simulink model "teach_from_joints"  (R2021a)
settings: Solver=FixedStepAuto  StartTime=0.0  StopTime=1000  FixedStep=SAMPLE_TIME  RelTol=1e-3
values from neighbouring files (symbols this model uses):
  dh_a = dh_list(:,3)    [move_joints_setup.m]
  dh_alpha = dh_list(:,4)    [move_joints_setup.m]
  dh_d = dh_list(:,2)+[0 0 0 0 0 length_f2t]'    [move_joints_setup.m]
  dh_theta_offset = dh_list(:,1)    [move_joints_setup.m]
  init_position = [274.5 0 543.1-138]    [move_joints_setup.m]
  initial_q = [0, 0, 0, 0, pi/2, 0]    [move_joints_setup.m]
  SAMPLE_TIME = 0.004    [move_joints_setup.m]
  theta_acc_max = theta_vel_max*2    [move_joints_setup.m]
  theta_max = [180,	80, 	70,     180,	110,	360]*pi/180    [move_joints_setup.m]
  theta_min = [-180,	-120,     -100,	-195,	-120,	-360]*pi/180    [move_joints_setup.m]
  theta_vel_max = [15, 10, 10, 40, 40, 40]*pi/180    [move_joints_setup.m]
undefined symbols (not defined in the file or in its folder): Px, Py, Pz, X, Y, Z
libraries: sm_lib x70, simulink x12, nesl_utility x11, dspswit3 x3, simulink_extras x2, sldrtlib x1, aerolibanimutils x1
(part 2 of 3)

== system teach_from_joints/Virtual_Robot_Subsystem/link_5 ==
  Inertia : sm_lib/Body Elements/Inertia  InertiaType=Custom  Mass=0.686166613628173  MassUnits=kg  CenterOfMass=[0, 0, 0]  CenterOfMassUnits=m  MomentsOfInertia=[0.00132263212499977, 0.000588220900408187, 0.00129230706392879]  MomentsOfInertiaUnits=kg*m^2  ProductsOfInertia=[9.33973775010868e-07, 6.88476103717453e-07, 5.90361537979662e-07]  ProductsOfInertiaUnits=kg*m^2  GraphicType=Marker  MarkerShape=Inertia  MarkerSize=20  GraphicVisPropType=SimpleVisualProperties  GraphicDiffuseColor=[0.5 0.5 0.5]  GraphicSpecularColor=[0.5 0.5 0.5 1.0]  GraphicAmbientColor=[0.15 0.15 0.15 1.0]  GraphicEmissiveColor=[0.0 0.0 0.0 1.0]  GraphicShininess=75  GraphicOpacity=1.0
  InertiaOriginTransform : sm_lib/Frames and Transforms/Rigid Transform  TranslationMethod=Cartesian  TranslationStandardOffset=0  TranslationLengthUnit=m  TranslationStandardAxis=+Z  TranslationCartesianOffset=[-0.0411790220693793, -0.0218038179681588, 5.10804574672119e-05]  TranslationROffset=0  TranslationROffsetUnits=m  TranslationZOffset=0  TranslationZOffsetUnits=m  TranslationThetaOffset=0  TranslationThetaOffsetUnits=deg  RotationMethod=RotationSequence  RotationAngleUnits=deg  RotationStandardAxis=+Z  RotationAngle=0.0  RotationArbitraryAxis=[0 0 1]  FollAlignAxisA=+X  BaseAlignAxisA=+Y  FollAlignAxisB=+Y  BaseAlignAxisB=+Z  RotationSequenceAxes=BaseAxes  RotationSequence=XYZ  RotationSequenceAngles=[0, 0, 0]  RotationSequenceAnglesUnits=rad  RotationMatrix=[1 0 0; 0 1 0; 0 0 1]
  ReferenceFrame : sm_lib/Frames and Transforms/Reference Frame
  Visual : sm_lib/Body Elements/File Solid  ExtGeomFileName=D:\matlab\tools\Mytool\Links-RT\MX\link_5.STL  UnitType=Custom  ExtGeomFileUnits=m  StepReaderType=HEX  ExportConvexHullGeometry=off  InertiaType=Custom  Mass=0  MassUnits=kg  CenterOfMass=[0, 0, 0]  CenterOfMassUnits=m  MomentsOfInertia=[0, 0, 0]  MomentsOfInertiaUnits=kg*m^2  ProductsOfInertia=[0, 0, 0]  ProductsOfInertiaUnits=kg*m^2  BasedOnType=Density  Density=1000  DensityUnits=kg/m^3  DoExposeReferenceFrame=on  SerializedFrames=<Frames/>  GraphicType=FromGeometry  MarkerShape=Sphere  MarkerSize=10  GraphicVisPropType=SimpleVisualProperties  GraphicDiffuseColor=[0.6 0.0 0.6]  GraphicSpecularColor=[0.5 0.5 0.5 1.0]  GraphicAmbientColor=[0.15 0.15 0.15 1.0]  GraphicEmissiveColor=[0.0 0.0 0.0 1.0]  GraphicShininess=75  GraphicOpacity=1
  VisualOriginTransform : sm_lib/Frames and Transforms/Rigid Transform  TranslationMethod=Cartesian  TranslationStandardOffset=0  TranslationLengthUnit=m  TranslationStandardAxis=+Z  TranslationCartesianOffset=[0, 0, 0]  TranslationROffset=0  TranslationROffsetUnits=m  TranslationZOffset=0  TranslationZOffsetUnits=m  TranslationThetaOffset=0  TranslationThetaOffsetUnits=deg  RotationMethod=RotationSequence  RotationAngleUnits=deg  RotationStandardAxis=+Z  RotationAngle=0.0  RotationArbitraryAxis=[0 0 1]  FollAlignAxisA=+X  BaseAlignAxisA=+Y  FollAlignAxisB=+Y  BaseAlignAxisB=+Z  RotationSequenceAxes=BaseAxes  RotationSequence=XYZ  RotationSequenceAngles=[0, 0, 0]  RotationSequenceAnglesUnits=rad  RotationMatrix=[1 0 0; 0 1 0; 0 0 1]
  joint_5_AxisInvTransform : sm_lib/Frames and Transforms/Rigid Transform  TranslationMethod=Cartesian  TranslationStandardOffset=0  TranslationLengthUnit=m  TranslationStandardAxis=+Z  TranslationCartesianOffset=[0, 0, 0]  TranslationROffset=0  TranslationROffsetUnits=m  TranslationZOffset=0  TranslationZOffsetUnits=m  TranslationThetaOffset=0  TranslationThetaOffsetUnits=deg  RotationMethod=ArbitraryAxis  RotationAngleUnits=rad  RotationStandardAxis=+Z  RotationAngle=1.571333286617217  RotationArbitraryAxis=[0.0006852597403183663, 0.9999996210465608, 0]  FollAlignAxisA=+X  BaseAlignAxisA=+Y  FollAlignAxisB=+Y  BaseAlignAxisB=+Z  RotationSequenceAxes=FollowerAxes  RotationSequence=XYX  RotationSequenceAngles=[0 0 0]  RotationSequenceAnglesUnits=deg  RotationMatrix=[1 0 0; 0 1 0; 0 0 1]
  joint_6_AxisTransform : sm_lib/Frames and Transforms/Rigid Transform  TranslationMethod=Cartesian  TranslationStandardOffset=0  TranslationLengthUnit=m  TranslationStandardAxis=+Z  TranslationCartesianOffset=[0, 0, 0]  TranslationROffset=0  TranslationROffsetUnits=m  TranslationZOffset=0  TranslationZOffsetUnits=m  TranslationThetaOffset=0  TranslationThetaOffsetUnits=deg  RotationMethod=ArbitraryAxis  RotationAngleUnits=rad  RotationStandardAxis=+Z  RotationAngle=1.569925857218851  RotationArbitraryAxis=[0.9999993866728818, -0.0006847895799997227, 0]  FollAlignAxisA=+X  BaseAlignAxisA=+Y  FollAlignAxisB=+Y  BaseAlignAxisB=+Z  RotationSequenceAxes=FollowerAxes  RotationSequence=XYX  RotationSequenceAngles=[0 0 0]  RotationSequenceAnglesUnits=deg  RotationMatrix=[1 0 0; 0 1 0; 0 0 1]
  joint_6_OriginTransform : sm_lib/Frames and Transforms/Rigid Transform  TranslationMethod=Cartesian  TranslationStandardOffset=0  TranslationLengthUnit=m  TranslationStandardAxis=+Z  TranslationCartesianOffset=[-0.041164, -0.10196, 6.9996e-05]  TranslationROffset=0  TranslationROffsetUnits=m  TranslationZOffset=0  TranslationZOffsetUnits=m  TranslationThetaOffset=0  TranslationThetaOffsetUnits=deg  RotationMethod=RotationSequence  RotationAngleUnits=deg  RotationStandardAxis=+Z  RotationAngle=0.0  RotationArbitraryAxis=[0 0 1]  FollAlignAxisA=+X  BaseAlignAxisA=+Y  FollAlignAxisB=+Y  BaseAlignAxisB=+Z  RotationSequenceAxes=BaseAxes  RotationSequence=XYZ  RotationSequenceAngles=[0, 0, 0]  RotationSequenceAnglesUnits=rad  RotationMatrix=[1 0 0; 0 1 0; 0 0 1]
  F : PMIOPort  Side=Left
  F1 : PMIOPort  Port=2  Side=Right
  connections:
  Inertia/RConn1 -- InertiaOriginTransform/RConn1
  ReferenceFrame/RConn1 -- InertiaOriginTransform/LConn1 -- joint_5_AxisInvTransform/LConn1 -- joint_6_OriginTransform/LConn1 -- VisualOriginTransform/LConn1
  Visual/RConn1 -- VisualOriginTransform/RConn1
  joint_5_AxisInvTransform/RConn1 -- F/RConn1
  joint_6_AxisTransform/RConn1 -- F1/RConn1
  joint_6_AxisTransform/LConn1 -- joint_6_OriginTransform/RConn1

== system teach_from_joints/Virtual_Robot_Subsystem/link_6 ==
  Inertia : sm_lib/Body Elements/Inertia  InertiaType=Custom  Mass=0.0837748471575824  MassUnits=kg  CenterOfMass=[0, 0, 0]  CenterOfMassUnits=m  MomentsOfInertia=[2.37096430738442e-05, 3.68399701824941e-05, 2.31857885737575e-05]  MomentsOfInertiaUnits=kg*m^2  ProductsOfInertia=[7.52372333523442e-08, 1.62958387540116e-10, 8.749655143078051e-09]  ProductsOfInertiaUnits=kg*m^2  GraphicType=Marker  MarkerShape=Inertia  MarkerSize=20  GraphicVisPropType=SimpleVisualProperties  GraphicDiffuseColor=[0.5 0.5 0.5]  GraphicSpecularColor=[0.5 0.5 0.5 1.0]  GraphicAmbientColor=[0.15 0.15 0.15 1.0]  GraphicEmissiveColor=[0.0 0.0 0.0 1.0]  GraphicShininess=75  GraphicOpacity=1.0
  InertiaOriginTransform : sm_lib/Frames and Transforms/Rigid Transform  TranslationMethod=Cartesian  TranslationStandardOffset=0  TranslationLengthUnit=m  TranslationStandardAxis=+Z  TranslationCartesianOffset=[-1.49769939650213e-05, -0.0138878614398256, -0.000131426803611889]  TranslationROffset=0  TranslationROffsetUnits=m  TranslationZOffset=0  TranslationZOffsetUnits=m  TranslationThetaOffset=0  TranslationThetaOffsetUnits=deg  RotationMethod=RotationSequence  RotationAngleUnits=deg  RotationStandardAxis=+Z  RotationAngle=0.0  RotationArbitraryAxis=[0 0 1]  FollAlignAxisA=+X  BaseAlignAxisA=+Y  FollAlignAxisB=+Y  BaseAlignAxisB=+Z  RotationSequenceAxes=BaseAxes  RotationSequence=XYZ  RotationSequenceAngles=[0, 0, 0]  RotationSequenceAnglesUnits=rad  RotationMatrix=[1 0 0; 0 1 0; 0 0 1]
  ReferenceFrame : sm_lib/Frames and Transforms/Reference Frame
  Visual : sm_lib/Body Elements/File Solid  ExtGeomFileName=D:\matlab\tools\Mytool\Links-RT\MX\link_6.STL  UnitType=Custom  ExtGeomFileUnits=m  StepReaderType=HEX  ExportConvexHullGeometry=off  InertiaType=Custom  Mass=0  MassUnits=kg  CenterOfMass=[0, 0, 0]  CenterOfMassUnits=m  MomentsOfInertia=[0, 0, 0]  MomentsOfInertiaUnits=kg*m^2  ProductsOfInertia=[0, 0, 0]  ProductsOfInertiaUnits=kg*m^2  BasedOnType=Density  Density=1000  DensityUnits=kg/m^3  DoExposeReferenceFrame=on  SerializedFrames=<Frames/>  GraphicType=FromGeometry  MarkerShape=Sphere  MarkerSize=10  GraphicVisPropType=SimpleVisualProperties  GraphicDiffuseColor=[1.0 0.4 0.0]  GraphicSpecularColor=[0.5 0.5 0.5 1.0]  GraphicAmbientColor=[0.15 0.15 0.15 1.0]  GraphicEmissiveColor=[0.0 0.0 0.0 1.0]  GraphicShininess=75  GraphicOpacity=1
  VisualOriginTransform : sm_lib/Frames and Transforms/Rigid Transform  TranslationMethod=Cartesian  TranslationStandardOffset=0  TranslationLengthUnit=m  TranslationStandardAxis=+Z  TranslationCartesianOffset=[0, 0, 0]  TranslationROffset=0  TranslationROffsetUnits=m  TranslationZOffset=0  TranslationZOffsetUnits=m  TranslationThetaOffset=0  TranslationThetaOffsetUnits=deg  RotationMethod=RotationSequence  RotationAngleUnits=deg  RotationStandardAxis=+Z  RotationAngle=0.0  RotationArbitraryAxis=[0 0 1]  FollAlignAxisA=+X  BaseAlignAxisA=+Y  FollAlignAxisB=+Y  BaseAlignAxisB=+Z  RotationSequenceAxes=BaseAxes  RotationSequence=XYZ  RotationSequenceAngles=[0, 0, 0]  RotationSequenceAnglesUnits=rad  RotationMatrix=[1 0 0; 0 1 0; 0 0 1]
  joint_6_AxisInvTransform : sm_lib/Frames and Transforms/Rigid Transform  TranslationMethod=Cartesian  TranslationStandardOffset=0  TranslationLengthUnit=m  TranslationStandardAxis=+Z  TranslationCartesianOffset=[0, 0, 0]  TranslationROffset=0  TranslationROffsetUnits=m  TranslationZOffset=0  TranslationZOffsetUnits=m  TranslationThetaOffset=0  TranslationThetaOffsetUnits=deg  RotationMethod=ArbitraryAxis  RotationAngleUnits=rad  RotationStandardAxis=+Z  RotationAngle=1.569925857218851  RotationArbitraryAxis=[0.9999993866728818, -0.0006847895799997227, 0]  FollAlignAxisA=+X  BaseAlignAxisA=+Y  FollAlignAxisB=+Y  BaseAlignAxisB=+Z  RotationSequenceAxes=FollowerAxes  RotationSequence=XYX  RotationSequenceAngles=[0 0 0]  RotationSequenceAnglesUnits=deg  RotationMatrix=[1 0 0; 0 1 0; 0 0 1]
  joint_tool0_OriginTransform : sm_lib/Frames and Transforms/Rigid Transform  TranslationMethod=Cartesian  TranslationStandardOffset=0  TranslationLengthUnit=m  TranslationStandardAxis=+Z  TranslationCartesianOffset=[0, -0.03183, 0]  TranslationROffset=0  TranslationROffsetUnits=m  TranslationZOffset=0  TranslationZOffsetUnits=m  TranslationThetaOffset=0  TranslationThetaOffsetUnits=deg  RotationMethod=RotationSequence  RotationAngleUnits=deg  RotationStandardAxis=+Z  RotationAngle=0.0  RotationArbitraryAxis=[0 0 1]  FollAlignAxisA=+X  BaseAlignAxisA=+Y  FollAlignAxisB=+Y  BaseAlignAxisB=+Z  RotationSequenceAxes=BaseAxes  RotationSequence=XYZ  RotationSequenceAngles=[0, 1.5707963268, 1.5707963268]  RotationSequenceAnglesUnits=rad  RotationMatrix=[1 0 0; 0 1 0; 0 0 1]
  F : PMIOPort  Side=Left
  F1 : PMIOPort  Port=2  Side=Right
  connections:
  Inertia/RConn1 -- InertiaOriginTransform/RConn1
  ReferenceFrame/RConn1 -- InertiaOriginTransform/LConn1 -- joint_6_AxisInvTransform/LConn1 -- joint_tool0_OriginTransform/LConn1 -- VisualOriginTransform/LConn1
  Visual/RConn1 -- VisualOriginTransform/RConn1
  joint_6_AxisInvTransform/RConn1 -- F/RConn1
  joint_tool0_OriginTransform/RConn1 -- F1/RConn1

== system teach_from_joints/Virtual_Robot_Subsystem/tool0 ==
  ReferenceFrame : sm_lib/Frames and Transforms/Reference Frame
  Rigid Transform : sm_lib/Frames and Transforms/Rigid Transform  TranslationMethod=Cartesian  TranslationStandardOffset=0  TranslationLengthUnit=m  TranslationStandardAxis=+Z  TranslationCartesianOffset=[0 0 0.136]  TranslationROffset=0  TranslationROffsetUnits=m  TranslationZOffset=0  TranslationZOffsetUnits=m  TranslationThetaOffset=0  TranslationThetaOffsetUnits=deg  RotationMethod=StandardAxis  RotationAngleUnits=deg  RotationStandardAxis=+X  RotationAngle=-90  RotationArbitraryAxis=[0 0 1]  FollAlignAxisA=+X  BaseAlignAxisA=+Y  FollAlignAxisB=+Y  BaseAlignAxisB=+Z  RotationSequenceAxes=FollowerAxes  RotationSequence=XYX  RotationSequenceAngles=[0 0 0]  RotationSequenceAnglesUnits=deg  RotationMatrix=[1 0 0; 0 1 0; 0 0 1]
  Visual : sm_lib/Body Elements/File Solid  ExtGeomFileName=D:\matlab\tools\Mytool\Links-RT\MX\tool.STEP  UnitType=FromFile  ExtGeomFileUnits=m  StepReaderType=HEX  ExportConvexHullGeometry=off  InertiaType=Custom  Mass=0  MassUnits=kg  CenterOfMass=[0, 0, 0]  CenterOfMassUnits=m  MomentsOfInertia=[0, 0, 0]  MomentsOfInertiaUnits=kg*m^2  ProductsOfInertia=[0, 0, 0]  ProductsOfInertiaUnits=kg*m^2  BasedOnType=Density  Density=1000  DensityUnits=kg/m^3  DoExposeReferenceFrame=on  SerializedFrames=<Frames/>  GraphicType=FromGeometry  MarkerShape=Sphere  MarkerSize=10  GraphicVisPropType=SimpleVisualProperties  GraphicDiffuseColor=[1.0 1.0 1.0]  GraphicSpecularColor=[0.5 0.5 0.5 1.0]  GraphicAmbientColor=[0.15 0.15 0.15 1.0]  GraphicEmissiveColor=[0.0 0.0 0.0 1.0]  GraphicShininess=75  GraphicOpacity=1
  VisualOriginTransform : sm_lib/Frames and Transforms/Rigid Transform  TranslationMethod=Cartesian  TranslationStandardOffset=0  TranslationLengthUnit=m  TranslationStandardAxis=+Z  TranslationCartesianOffset=[0, 0, 0]  TranslationROffset=0  TranslationROffsetUnits=m  TranslationZOffset=0  TranslationZOffsetUnits=m  TranslationThetaOffset=0  TranslationThetaOffsetUnits=deg  RotationMethod=RotationSequence  RotationAngleUnits=deg  RotationStandardAxis=+Z  RotationAngle=0.0  RotationArbitraryAxis=[0 0 1]  FollAlignAxisA=+X  BaseAlignAxisA=+Y  FollAlignAxisB=+Y  BaseAlignAxisB=+Z  RotationSequenceAxes=BaseAxes  RotationSequence=XYZ  RotationSequenceAngles=[-90, 0, 0]  RotationSequenceAnglesUnits=deg  RotationMatrix=[1 0 0; 0 1 0; 0 0 1]
  F : PMIOPort  Side=Left
  connections:
  ReferenceFrame/RConn1 -- F/RConn1 -- VisualOriginTransform/LConn1
  Visual/RConn1 -- VisualOriginTransform/RConn1

== system teach_from_joints/traj_planing/Enabled Subsystem1 ==
  In1 : Inport
  Enable : EnablePort
  Out1 : Outport
  wires:
  In1/1 -> Out1/1

== system teach_from_joints/traj_planing/Subsystem ==
  In1 : Inport
  Enable : EnablePort
  Gain1 : Gain
  Out1 : Outport
  wires:
  Gain1/1 -> Out1/1
  In1/1 -> Gain1/1

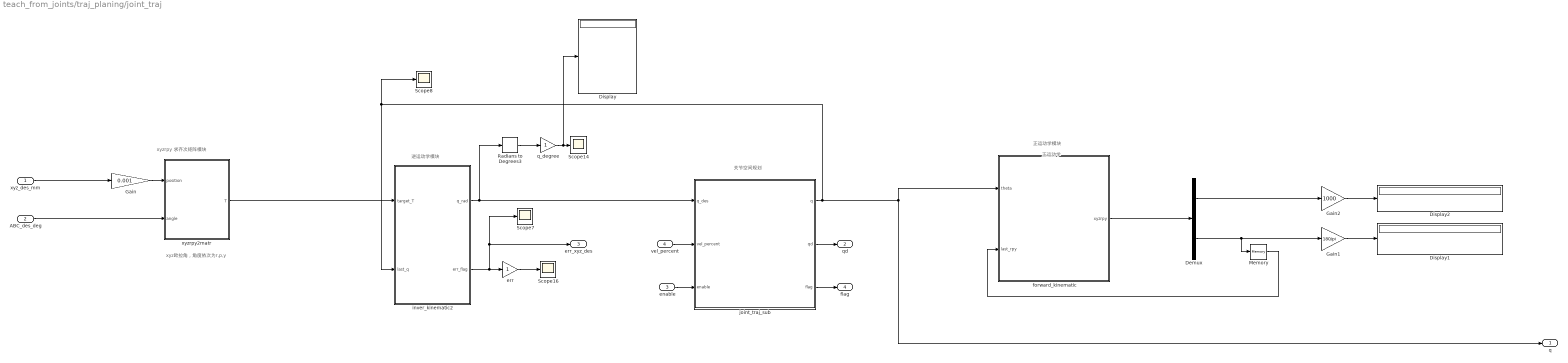
== system teach_from_joints/traj_planing/joint_traj ==
  note: xyz欧拉角，角度依次为r,p,y
  note: 逆运动学模块
  note: 关节空间规划
  note: xyzrpy 求齐次矩阵模块
  note: 正运动学
  note: 正运动学模块
  xyz_des_mm : Inport
  ABC_des_deg : Inport  Port=2
  enable : Inport  Port=3
  vel_percent : Inport  Port=4
  Demux : Demux  Outputs=2
  Display : Display
  Display1 : Display
  Display2 : Display
  Gain : Gain  Gain=0.001
  Gain1 : Gain  Gain=180/pi
  Gain2 : Gain  Gain=1000
  Memory : Memory
  Radians to Degrees3 : simulink_extras/Transformations/Radians to Degrees
  Scope{7..8,14,16} (4 alike) : Scope
  err : Gain
  forward_kinematic : Subsystem
  inver_kinematic2 : Subsystem
  joint_traj_sub : Subsystem
  q_degree : Gain
  xyzrpy2matr : MATLAB Function  TreatAsAtomicUnit=on
  q : Outport
  qd : Outport  Port=2
  err_xyz_des : Outport  Port=3
  flag : Outport  Port=4
  wires:
  inver_kinematic2/1(q_rad) -> joint_traj_sub/1(q_des), Radians to Degrees3/1
  inver_kinematic2/2(err_flag) -> err_xyz_des/1, Scope7/1, err/1
  q_degree/1 -> Display/1, Scope14/1
  Radians to Degrees3/1 -> q_degree/1
  err/1 -> Scope16/1
  vel_percent/1 -> joint_traj_sub/2(vel_percent)
  enable/1 -> joint_traj_sub/3(enable)
  joint_traj_sub/2(qd) -> qd/1
  xyzrpy2matr/1(T) -> inver_kinematic2/1(target_T)
  ABC_des_deg/1 -> xyzrpy2matr/2(angle)
  xyz_des_mm/1 -> Gain/1
  Gain/1 -> xyzrpy2matr/1(position)
  joint_traj_sub/3(flag) -> flag/1
  Demux/2 -> Gain1/1, Memory/1
  Gain1/1 -> Display1/1
  Gain2/1 -> Display2/1
  Demux/1 -> Gain2/1
  joint_traj_sub/1(q) -> forward_kinematic/1(theta), q/1, Scope8/1, inver_kinematic2/2(last_q)
  forward_kinematic/1(xyzrpy) -> Demux/1
  Memory/1 -> forward_kinematic/2(last_rpy)

== system teach_from_joints/traj_planing/zeros_vel_check ==
  q : Inport
  Abs : Abs
  Compare To Zero : simulink/Logic and Bit Operations/Compare To Zero  relop===  OutDataTypeStr=boolean
  Dead Zone : DeadZone  LowerValue=0  UpperValue=0.001  SaturateOnIntegerOverflow=on
  Difference : simulink/Discrete/Difference  ICPrevInput=initial_q  OutMin=[]  OutMax=[]  OutDataType=fixdt(1, 16)  OutScaling=2^-10  DoSatur=off
  Memory1 : Memory  InitialCondition=1  InheritSampleTime=on
  Scope15 : Scope
  Scope16 : Scope
  Scope9 : Scope
  Sum of Elements : Sum  Inputs=+
  change_flag : Outport
  wires:
  q/1 -> Difference/1
  Abs/1 -> Sum of Elements/1
  Dead Zone/1 -> Compare To Zero/1, Scope16/1
  Memory1/1 -> change_flag/1, Scope15/1
  Difference/1 -> Scope9/1, Abs/1
  Compare To Zero/1 -> Memory1/1
  Sum of Elements/1 -> Dead Zone/1

== system teach_from_joints/traj_planing/joint_traj/forward_kinematic ==
  theta : Inport
  last_rpy : Inport  Port=2
  Constant : Constant  Value=dh_theta_offset
  Constant1 : Constant  Value=dh_d
  Constant2 : Constant  Value=dh_a
  Constant3 : Constant  Value=dh_alpha
  MATLAB Function : MATLAB Function  TreatAsAtomicUnit=on
  MATLAB Function1 : MATLAB Function  TreatAsAtomicUnit=on
  xyzrpy : Outport
  wires:
  Constant3/1 -> MATLAB Function/5(alpha)
  MATLAB Function/1(T) -> MATLAB Function1/1(T)
  Constant2/1 -> MATLAB Function/4(a)
  Constant1/1 -> MATLAB Function/3(d)
  Constant/1 -> MATLAB Function/2(theta_offset)
  theta/1 -> MATLAB Function/1(theta)
  last_rpy/1 -> MATLAB Function1/2(last_rpy)
  MATLAB Function1/1(xyzrpy) -> xyzrpy/1

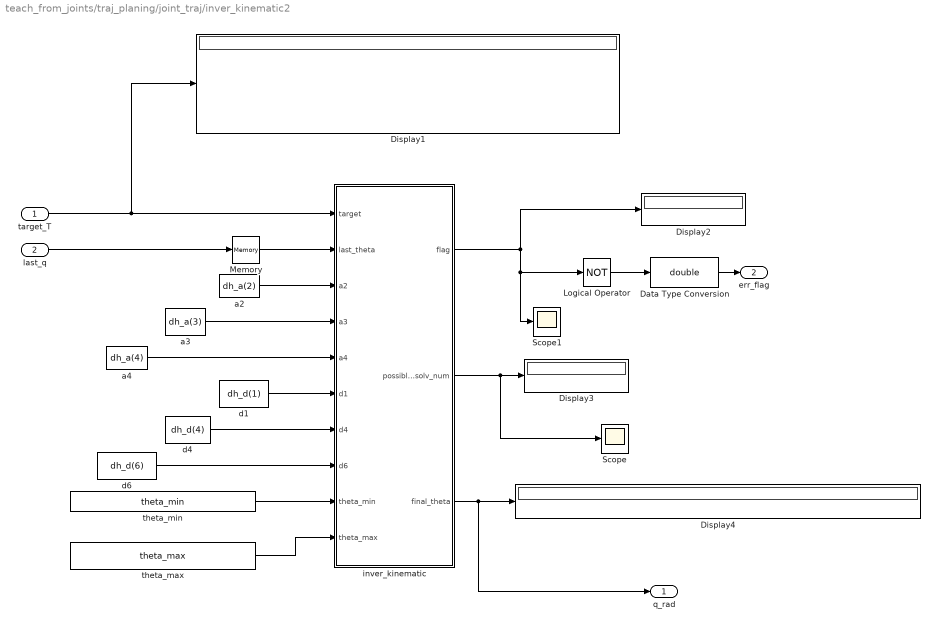
== system teach_from_joints/traj_planing/joint_traj/inver_kinematic2 ==
  target_T : Inport
  last_q : Inport  Port=2
  Data Type Conversion : DataTypeConversion  OutDataTypeStr=double
  Display{1..4} (4 alike) : Display
  Logical Operator : Logic  Operator=NOT  AllPortsSameDT=off  OutDataTypeStr=boolean
  Memory : Memory  InitialCondition=initial_q  InheritSampleTime=on
  Scope : Scope
  Scope1 : Scope
  a2 : Constant  Value=dh_a(2)
  a3 : Constant  Value=dh_a(3)
  a4 : Constant  Value=dh_a(4)
  d1 : Constant  Value=dh_d(1)
  d4 : Constant  Value=dh_d(4)
  d6 : Constant  Value=dh_d(6)
  inver_kinematic : MATLAB Function  TreatAsAtomicUnit=on
  theta_max : Constant  Value=theta_max
  theta_min : Constant  Value=theta_min
  q_rad : Outport
  err_flag : Outport  Port=2
  wires:
  inver_kinematic/1(flag) -> Logical Operator/1, Scope1/1, Display2/1
  inver_kinematic/2(possible_solv_num) -> Scope/1, Display3/1
  d6/1 -> inver_kinematic/8(d6)
  d1/1 -> inver_kinematic/6(d1)
  target_T/1 -> Display1/1, inver_kinematic/1(target)
  theta_max/1 -> inver_kinematic/10(theta_max)
  a3/1 -> inver_kinematic/4(a3)
  a4/1 -> inver_kinematic/5(a4)
  a2/1 -> inver_kinematic/3(a2)
  d4/1 -> inver_kinematic/7(d4)
  Memory/1 -> inver_kinematic/2(last_theta)
  theta_min/1 -> inver_kinematic/9(theta_min)
  Logical Operator/1 -> Data Type Conversion/1
  Data Type Conversion/1 -> err_flag/1
  inver_kinematic/3(final_theta) -> q_rad/1, Display4/1
  last_q/1 -> Memory/1

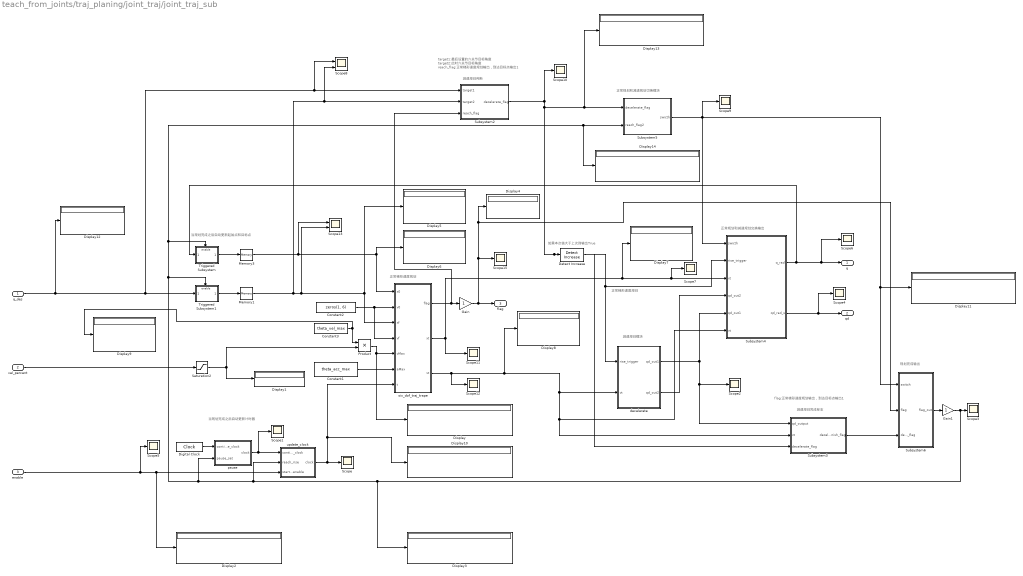
== system teach_from_joints/traj_planing/joint_traj/joint_traj_sub ==
  note: 当规划完成之后自动更新起始点和目标点
  note: 正常梯形速度规划
  note: 减速规划判断
  note: 正常规划和减速规划切换模块
  note: 规划完成输出
  note: 减速规划完成标志
  note: 正常规划和减速规划交换输出
  note: 减速规划模块
  note: 当规划完成之后自动更新计时器
  note: 正常梯形速度规划
  note: flag:正常梯形速度规划输出，到达目标点输出1
  note: target1:最后设置的六关节目标角度
      | target2:此时六关节目标角度
      | reach_flag:正常梯形速度规划输出，到达目标点输出1
  note: 如果本次值大于上次则输出True
  q_des : Inport
  vel_percent : Inport  Port=2
  enable : Inport  Port=3
  Constant1 : Constant  Value=theta_acc_max
  Constant2 : Constant  Value=zeros(1, 6)
  Constant3 : Constant  Value=theta_vel_max
  Detect Increase : simulink/Logic and Bit Operations/Detect Increase  vinit=0.0  OutDataTypeStr=boolean
  Digital Clock : DigitalClock  SampleTime=SAMPLE_TIME
  Display{,1..14} (15 alike) : Display
  Gain : Gain
  Gain1 : Gain
  Memory1 : Memory  InitialCondition=initial_q  InheritSampleTime=on
  Memory3 : Memory  InitialCondition=initial_q  InheritSampleTime=on
  Product : Product
  Saturation2 : Saturate  UpperLimit=1  LowerLimit=0.01
  Scope{,1..7,9..12,15} (13 alike) : Scope
  Scope13 : Scope  NumInputPorts=2
  Scope8 : Scope  NumInputPorts=2
  Subsystem2 : Subsystem
  Subsystem3 : Subsystem
  Subsystem4 : Subsystem
  Subsystem5 : Subsystem
  Subsystem6 : Subsystem
  Triggered Subsystem : Subsystem  TreatAsAtomicUnit=on
  Triggered Subsystem1 : Subsystem  TreatAsAtomicUnit=on
  decelerate : Subsystem
  pause : Subsystem
  six_dof_traj_trape : MATLAB Function  TreatAsAtomicUnit=on
  update_clock : Subsystem
  q : Outport
  qd : Outport  Port=2
  flag : Outport  Port=3
  wires:
  q_des/1 -> Display12/1, Scope8/1, Subsystem2/1(target1), Triggered Subsystem1/1(q_des)
  Constant2/1 -> six_dof_traj_trape/4(vf), six_dof_traj_trape/2(v0)
  Digital Clock/1 -> pause/1(continue_clock)
  Memory3/1 -> Scope13/1, Display6/1, six_dof_traj_trape/1(x0)
  enable/1 -> Scope5/1, Display2/1, update_clock/3(start_enable)
  update_clock/1(clock) -> six_dof_traj_trape/7(t), Display10/1, Scope/1
  pause/1(clock) -> update_clock/1(continue_clock), Scope1/1
  Subsystem3/1(decelerate_finish_flag) -> Subsystem6/3(decelerate_flag)
  Triggered Subsystem/1(Out1) -> Memory3/1
  Gain1/1 -> Display3/1, pause/2(pause_set), Triggered Subsystem/Enable, Display14/1, Subsystem5/2(reach_flag2), Triggered Subsystem1/Enable, update_clock/2(reach_rise), Scope3/1
  Subsystem6/1(flag_out) -> Gain1/1
  Constant3/1 -> Product/1, Display9/1
  Subsystem4/2(qd_rad_s) -> Scope4/1, qd/1
  Triggered Subsystem1/1(Out1) -> Memory1/1
  six_dof_traj_trape/3(vt) -> Scope12/1, Display8/1, Subsystem4/6(vt), Subsystem3/2(vt), decelerate/2(vt)
  Saturation2/1 -> Display1/1, Product/2
  Detect Increase/1 -> decelerate/1(rise_trigger), Subsystem4/2(rise_trigger)
  six_dof_traj_trape/2(xt) -> Scope7/1, Subsystem4/3(xt), Display7/1, Scope11/1
  Gain/1 -> flag/1, Subsystem6/2(flag), Display4/1, Scope15/1
  Subsystem4/1(q_rad) -> Triggered Subsystem/1(q_rad), Scope6/1, q/1
  Subsystem2/1(decelerate_flag) -> Display13/1, Subsystem5/1(decelerate_flag), Subsystem3/3(decelerate_flag), Detect Increase/1, Scope10/1
  decelerate/1(qd_out1) -> Subsystem4/5(qd_out1), Subsystem3/1(qd_output), Scope2/1
  decelerate/2(qd_out2) -> Subsystem4/4(qd_out2)
  vel_percent/1 -> Saturation2/1
  Product/1 -> Display/1, six_dof_traj_trape/5(vMax)
  six_dof_traj_trape/1(flag) -> Gain/1, Subsystem2/3(reach_flag)
  Subsystem5/1(swicth) -> Subsystem4/1(swicth), Display11/1, Subsystem6/1(switch), Scope9/1
  Constant1/1 -> six_dof_traj_trape/6(aMax)
  Memory1/1 -> Scope8/2, Subsystem2/2(target2), Scope13/2, Display5/1, six_dof_traj_trape/3(xf)

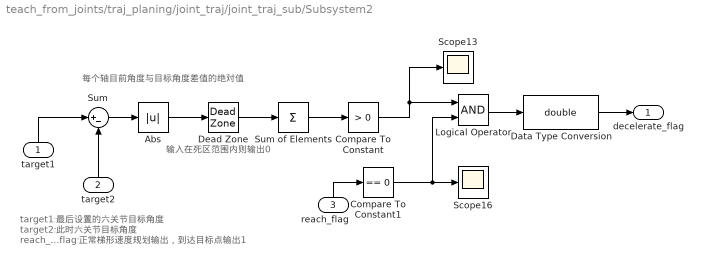
== system teach_from_joints/traj_planing/joint_traj/joint_traj_sub/Subsystem2 ==
  note: 每个轴目前角度与目标角度差值的绝对值
  note: 输入在死区范围内则输出0
  note: target1:最后设置的六关节目标角度
      | target2:此时六关节目标角度
      | reach_flag:正常梯形速度规划输出，到达目标点输出1
  target1 : Inport
  target2 : Inport  Port=2
  reach_flag : Inport  Port=3
  Abs : Abs
  Compare To Constant : simulink/Logic and Bit Operations/Compare To Constant  relop=>  const=0  OutDataTypeStr=boolean
  Compare To Constant1 : simulink/Logic and Bit Operations/Compare To Constant  relop===  const=0  OutDataTypeStr=boolean
  Data Type Conversion : DataTypeConversion  OutDataTypeStr=double
  Dead Zone : DeadZone  LowerValue=0  UpperValue=0.0001*ones(1,6)  SaturateOnIntegerOverflow=on
  Logical Operator : Logic  AllPortsSameDT=off  OutDataTypeStr=boolean
  Scope13 : Scope
  Scope16 : Scope
  Sum : Sum  Inputs=|+-
  Sum of Elements : Sum  Inputs=+
  decelerate_flag : Outport
  wires:
  target1/1 -> Sum/1
  target2/1 -> Sum/2
  reach_flag/1 -> Compare To Constant1/1
  Compare To Constant/1 -> Logical Operator/1, Scope13/1
  Logical Operator/1 -> Data Type Conversion/1
  Sum of Elements/1 -> Compare To Constant/1
  Dead Zone/1 -> Sum of Elements/1
  Compare To Constant1/1 -> Scope16/1, Logical Operator/2
  Data Type Conversion/1 -> decelerate_flag/1
  Sum/1 -> Abs/1
  Abs/1 -> Dead Zone/1

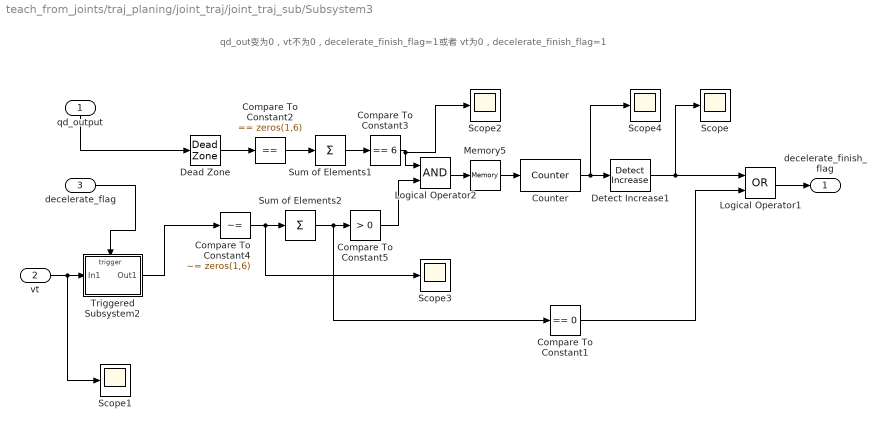
== system teach_from_joints/traj_planing/joint_traj/joint_traj_sub/Subsystem3 ==
  note: qd_out变为0，vt不为0，decelerate_finish_flag=1
      | 或者 vt为0，decelerate_finish_flag=1
  qd_output : Inport
  vt : Inport  Port=2
  decelerate_flag : Inport  Port=3
  Compare To Constant1 : simulink/Logic and Bit Operations/Compare To Constant  relop===  const=0  OutDataTypeStr=boolean
  Compare To Constant2 : simulink/Logic and Bit Operations/Compare To Constant  relop===  const=zeros(1,6)  OutDataTypeStr=boolean
  Compare To Constant3 : simulink/Logic and Bit Operations/Compare To Constant  relop===  const=6  OutDataTypeStr=boolean
  Compare To Constant4 : simulink/Logic and Bit Operations/Compare To Constant  relop=~=  const=zeros(1,6)  OutDataTypeStr=boolean
  Compare To Constant5 : simulink/Logic and Bit Operations/Compare To Constant  relop=>  const=0  OutDataTypeStr=boolean
  Counter : dspswit3/Counter  Direction=Up  CountEvent=Non-zero sample  CounterSize=User defined  MaxCount=1  InitialCount=0  Output=Count  HitValue=32  ResetInput=off  SamplesPerFrame=1  Ts=1  CntDtype=double  HitDtype=Logical
  Dead Zone : DeadZone  LowerValue=-theta_acc_max*SAMPLE_TIME*1.5  UpperValue=theta_acc_max*SAMPLE_TIME*1.5  SaturateOnIntegerOverflow=on
  Detect Increase1 : simulink/Logic and Bit Operations/Detect Increase  vinit=0.0  OutDataTypeStr=boolean
  Logical Operator1 : Logic  Operator=OR  AllPortsSameDT=off  OutDataTypeStr=boolean
  Logical Operator2 : Logic  AllPortsSameDT=off  OutDataTypeStr=boolean
  Memory5 : Memory  InheritSampleTime=on
  Scope{,1..4} (5 alike) : Scope
  Sum of Elements1 : Sum  Inputs=+
  Sum of Elements2 : Sum  Inputs=+
  Triggered Subsystem2 : Subsystem  TreatAsAtomicUnit=on
  decelerate_finish_flag : Outport
  wires:
  qd_output/1 -> Dead Zone/1
  Compare To Constant2/1 -> Sum of Elements1/1
  Sum of Elements1/1 -> Compare To Constant3/1
  Dead Zone/1 -> Compare To Constant2/1
  Logical Operator2/1 -> Memory5/1
  Memory5/1 -> Counter/1
  Compare To Constant4/1 -> Scope3/1, Sum of Elements2/1
  Sum of Elements2/1 -> Compare To Constant1/1, Compare To Constant5/1
  Compare To Constant5/1 -> Logical Operator2/2
  Triggered Subsystem2/1(Out1) -> Compare To Constant4/1
  Compare To Constant3/1 -> Scope2/1, Logical Operator2/1
  Detect Increase1/1 -> Logical Operator1/1, Scope/1
  decelerate_flag/1 -> Triggered Subsystem2/Trigger
  vt/1 -> Scope1/1, Triggered Subsystem2/1(In1)
  Counter/1 -> Scope4/1, Detect Increase1/1
  Logical Operator1/1 -> decelerate_finish_flag/1
  Compare To Constant1/1 -> Logical Operator1/2

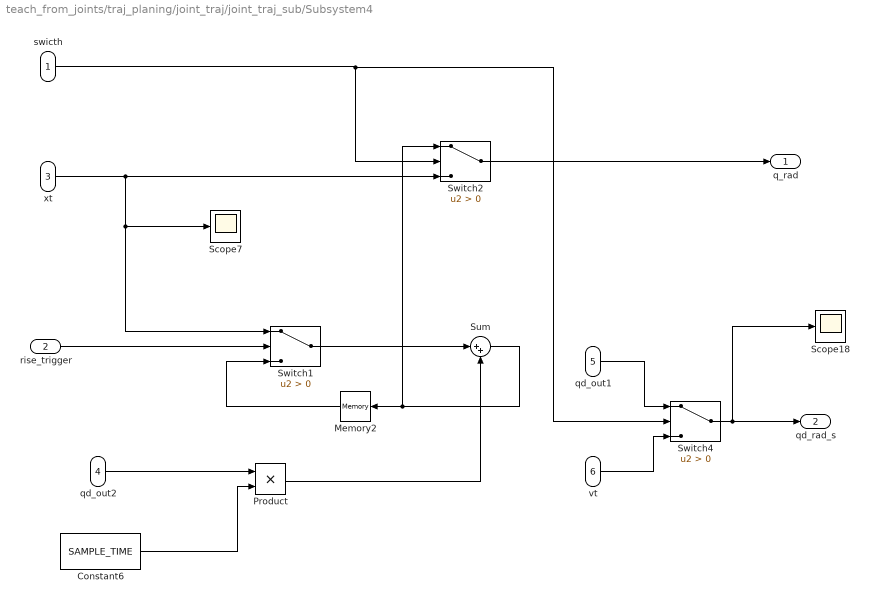
== system teach_from_joints/traj_planing/joint_traj/joint_traj_sub/Subsystem4 ==
  swicth : Inport
  rise_trigger : Inport  Port=2
  xt : Inport  Port=3
  qd_out2 : Inport  Port=4
  qd_out1 : Inport  Port=5
  vt : Inport  Port=6
  Constant6 : Constant  Value=SAMPLE_TIME
  Memory2 : Memory  InitialCondition=initial_q  InheritSampleTime=on
  Product : Product
  Scope18 : Scope
  Scope7 : Scope
  Sum : Sum  Inputs=|++
  Switch1 : Switch  Criteria=u2 > Threshold
  Switch2 : Switch  Criteria=u2 > Threshold
  Switch4 : Switch  Criteria=u2 > Threshold
  q_rad : Outport
  qd_rad_s : Outport  Port=2
  wires:
  vt/1 -> Switch4/3
  rise_trigger/1 -> Switch1/2
  swicth/1 -> Switch4/2, Switch2/2
  xt/1 -> Switch1/1, Scope7/1, Switch2/3
  qd_out2/1 -> Product/1
  qd_out1/1 -> Switch4/1
  Switch1/1 -> Sum/1
  Sum/1 -> Switch2/1, Memory2/1
  Memory2/1 -> Switch1/3
  Constant6/1 -> Product/2
  Product/1 -> Sum/2
  Switch4/1 -> qd_rad_s/1, Scope18/1
  Switch2/1 -> q_rad/1

== system teach_from_joints/traj_planing/joint_traj/joint_traj_sub/Subsystem5 ==
  note: Inc和Rst都是上升沿触发，Inc的优先级高
  decelerate_flag : Inport
  reach_flag2 : Inport  Port=2
  Counter : dspswit3/Counter  Direction=Up  CountEvent=Rising edge  CounterSize=User defined  MaxCount=1  InitialCount=0  Output=Count  HitValue=32  ResetInput=on  SamplesPerFrame=1  Ts=1  CntDtype=double  HitDtype=Logical
  Display1 : Display
  Display11 : Display
  Memory7 : Memory  InheritSampleTime=on
  Scope9 : Scope
  swicth : Outport
  wires:
  reach_flag2/1 -> Memory7/1
  decelerate_flag/1 -> Display1/1, Counter/1
  Counter/1 -> swicth/1
  Memory7/1 -> Counter/2, Scope9/1, Display11/1

== system teach_from_joints/traj_planing/joint_traj/joint_traj_sub/Subsystem6 ==
  switch : Inport
  flag : Inport  Port=2
  decelerate_flag : Inport  Port=3
  Delay : Delay  DelayLength=1  InitialCondition=1
  Scope17 : Scope
  Scope8 : Scope
  Switch3 : Switch  Criteria=u2 > Threshold
  flag_out : Outport
  wires:
  decelerate_flag/1 -> Switch3/1, Scope8/1
  Switch3/1 -> Delay/1
  flag/1 -> Scope17/1, Switch3/3
  switch/1 -> Switch3/2
  Delay/1 -> flag_out/1

== system teach_from_joints/traj_planing/joint_traj/joint_traj_sub/Triggered Subsystem ==
  q_rad : Inport
  Enable : EnablePort
  Out1 : Outport
  wires:
  q_rad/1 -> Out1/1

== system teach_from_joints/traj_planing/joint_traj/joint_traj_sub/Triggered Subsystem1 ==
  q_des : Inport
  Enable : EnablePort
  Out1 : Outport
  wires:
  q_des/1 -> Out1/1

== system teach_from_joints/traj_planing/joint_traj/joint_traj_sub/decelerate ==
  note: decelerate_flag从0变为1，rise_trigger在一个SAMPLE_TIME内为1
  rise_trigger : Inport
  vt : Inport  Port=2
  Constant : Constant  Value=SAMPLE_TIME
  Constant3 : Constant  Value=theta_vel_max
  Constant4 : Constant  Value=theta_acc_max
  Constant5 : Constant  Value=zeros(1,6)
  Memory : Memory  InitialCondition=zeros(1,6)  InheritSampleTime=on
  Scope5 : Scope
  Switch : Switch  Criteria=u2 > Threshold
  Terminator : Terminator
  limit_qd : MATLAB Function  TreatAsAtomicUnit=on
  qd_out1 : Outport
  qd_out2 : Outport  Port=2
  wires:
  Memory/1 -> qd_out2/1, Switch/3
  Constant/1 -> limit_qd/5(dt)
  limit_qd/2(percent_min) -> Terminator/1
  Constant3/1 -> limit_qd/3(qd_max)
  Constant4/1 -> limit_qd/4(qdd_max)
  Switch/1 -> limit_qd/2(last_qd)
  Constant5/1 -> limit_qd/1(qd_input)
  rise_trigger/1 -> Switch/2
  vt/1 -> Switch/1
  limit_qd/1(qd_output) -> Memory/1, Scope5/1, qd_out1/1

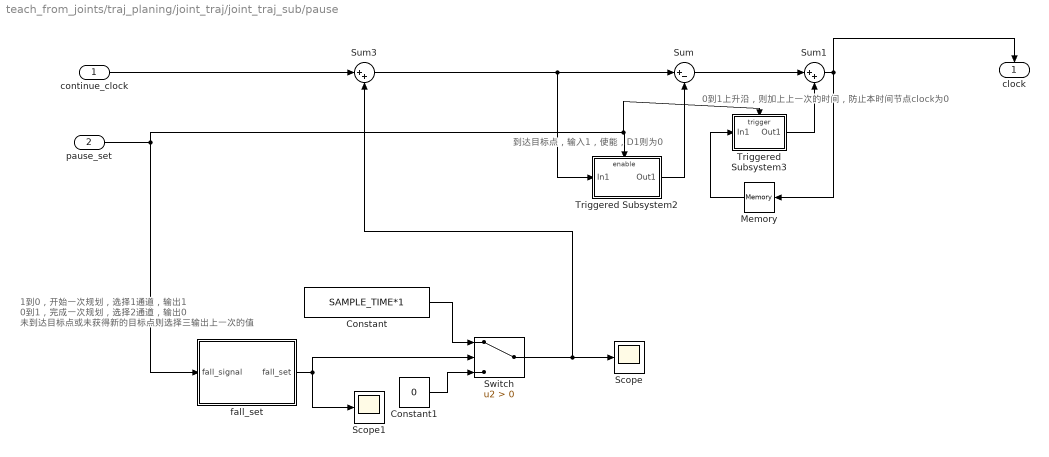
== system teach_from_joints/traj_planing/joint_traj/joint_traj_sub/pause ==
  note: 到达目标点，输入1，使能，D1则为0
  note: 1到0，开始一次规划，选择1通道，输出1
      | 0到1，完成一次规划，选择2通道，输出0
      | 未到达目标点或未获得新的目标点则选择三输出上一次的值
  note: 0到1上升沿，则加上上一次的时间，防止本时间节点clock为0
  continue_clock : Inport
  pause_set : Inport  Port=2
  Constant : Constant  Value=SAMPLE_TIME*1
  Constant1 : Constant  Value=0
  Memory : Memory  InheritSampleTime=on
  Scope : Scope
  Scope1 : Scope
  Sum : Sum  Inputs=|+-
  Sum1 : Sum  Inputs=|++
  Sum3 : Sum  Inputs=|++
  Switch : Switch  Criteria=u2 > Threshold
  Triggered Subsystem2 : Subsystem  TreatAsAtomicUnit=on
  Triggered Subsystem3 : Subsystem  TreatAsAtomicUnit=on
  fall_set : Subsystem
  clock : Outport
  wires:
  pause_set/1 -> Triggered Subsystem3/Trigger, Triggered Subsystem2/Enable, fall_set/1(fall_signal)
  Sum/1 -> Sum1/1
  Triggered Subsystem2/1(Out1) -> Sum/2
  Memory/1 -> Triggered Subsystem3/1(In1)
  Sum3/1 -> Triggered Subsystem2/1(In1), Sum/1
  Triggered Subsystem3/1(Out1) -> Sum1/2
  Constant/1 -> Switch/1
  Switch/1 -> Sum3/2, Scope/1
  Constant1/1 -> Switch/3
  Sum1/1 -> clock/1, Memory/1
  fall_set/1(fall_set) -> Scope1/1, Switch/2
  continue_clock/1 -> Sum3/1

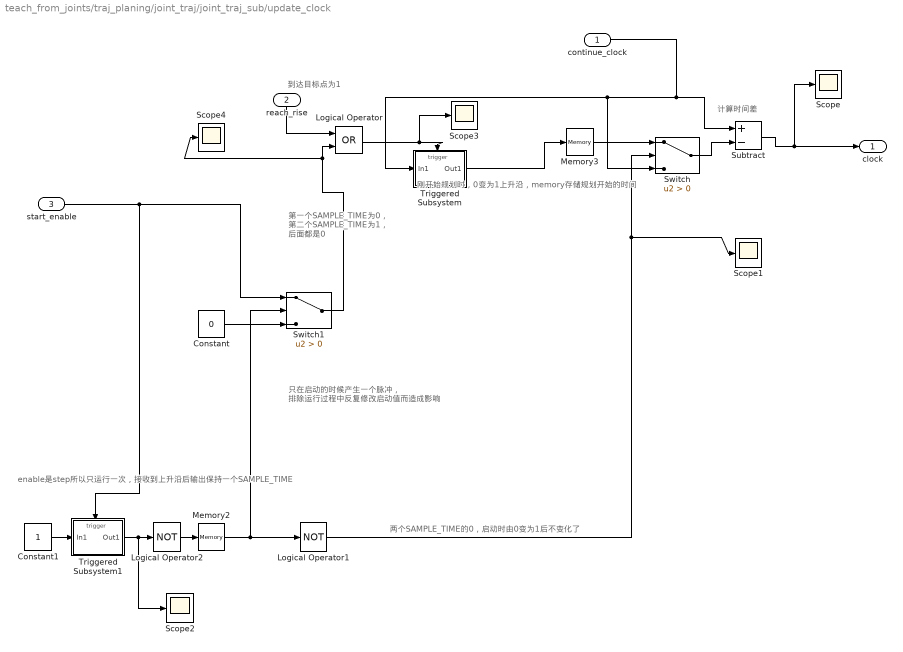
== system teach_from_joints/traj_planing/joint_traj/joint_traj_sub/update_clock ==
  note: 第一个SAMPLE_TIME为0，
      | 第二个SAMPLE_TIME为1，
      | 后面都是0
  note: enable是step所以只运行一次，接收到上升沿后输出保持一个SAMPLE_TIME
  note: 只在启动的时候产生一个脉冲，
      | 排除运行过程中反复修改启动值而造成影响
  note: 到达目标点为1
  note: 刚开始规划时，0变为1上升沿，memory存储规划开始的时间
  note: 两个SAMPLE_TIME的0，启动时由0变为1后不变化了
  note: 计算时间差
  continue_clock : Inport
  reach_rise : Inport  Port=2
  start_enable : Inport  Port=3
  Constant : Constant  Value=0
  Constant1 : Constant
  Logical Operator : Logic  Operator=OR  AllPortsSameDT=off  OutDataTypeStr=boolean
  Logical Operator1 : Logic  Operator=NOT  AllPortsSameDT=off  OutDataTypeStr=boolean
  Logical Operator2 : Logic  Operator=NOT  AllPortsSameDT=off  OutDataTypeStr=boolean
  Memory2 : Memory  InitialCondition=1  InheritSampleTime=on
  Memory3 : Memory  InheritSampleTime=on
  Scope{,1..4} (5 alike) : Scope
  Subtract : Sum  Inputs=+-
  Switch : Switch  Criteria=u2 > Threshold
  Switch1 : Switch  Criteria=u2 > Threshold
  Triggered Subsystem : Subsystem  TreatAsAtomicUnit=on
  Triggered Subsystem1 : Subsystem  TreatAsAtomicUnit=on
  clock : Outport
  wires:
  Memory3/1 -> Switch/1
  continue_clock/1 -> Switch/3, Triggered Subsystem/1(In1), Subtract/1
  reach_rise/1 -> Logical Operator/1
  Subtract/1 -> Scope/1, clock/1
  Triggered Subsystem/1(Out1) -> Memory3/1
  Switch/1 -> Subtract/2
  Logical Operator/1 -> Scope3/1, Triggered Subsystem/Trigger
  start_enable/1 -> Triggered Subsystem1/Trigger, Switch1/1
  Switch1/1 -> Scope4/1, Logical Operator/2
  Triggered Subsystem1/1(Out1) -> Logical Operator2/1, Scope2/1
  Memory2/1 -> Switch1/2, Logical Operator1/1
  Constant/1 -> Switch1/3
  Logical Operator1/1 -> Scope1/1, Switch/2
  Constant1/1 -> Triggered Subsystem1/1(In1)
  Logical Operator2/1 -> Memory2/1

== system teach_from_joints/traj_planing/joint_traj/joint_traj_sub/Subsystem3/Triggered Subsystem2 ==
  In1 : Inport
  Trigger : TriggerPort  VariantControl=Variant  PortDimensions=1
  Out1 : Outport
  wires:
  In1/1 -> Out1/1

== system teach_from_joints/traj_planing/joint_traj/joint_traj_sub/pause/Triggered Subsystem2 ==
  In1 : Inport
  Enable : EnablePort
  Out1 : Outport
  wires:
  In1/1 -> Out1/1

== system teach_from_joints/traj_planing/joint_traj/joint_traj_sub/pause/Triggered Subsystem3 ==
  In1 : Inport
  Trigger : TriggerPort  VariantControl=Variant
  Out1 : Outport
  wires:
  In1/1 -> Out1/1

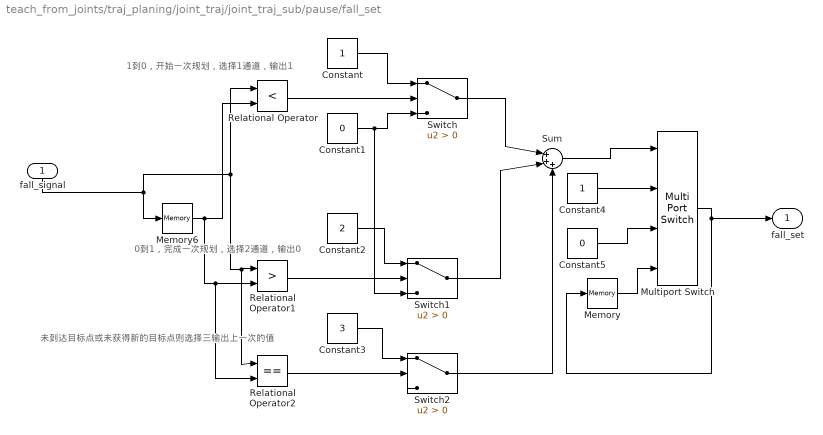
== system teach_from_joints/traj_planing/joint_traj/joint_traj_sub/pause/fall_set ==
  note: 0到1，完成一次规划，选择2通道，输出0
  note: 1到0，开始一次规划，选择1通道，输出1
  note: 未到达目标点或未获得新的目标点则选择三输出上一次的值
  fall_signal : Inport
  Constant : Constant
  Constant1 : Constant  Value=0
  Constant2 : Constant  Value=2
  Constant3 : Constant  Value=3
  Constant4 : Constant
  Constant5 : Constant  Value=0
  Memory : Memory  InheritSampleTime=on
  Memory6 : Memory  InheritSampleTime=on
  Multiport Switch : MultiPortSwitch
  Relational Operator : RelationalOperator  Operator=<  OutDataTypeStr=boolean  RndMeth=Simplest
  Relational Operator1 : RelationalOperator  Operator=>  OutDataTypeStr=boolean  RndMeth=Simplest
  Relational Operator2 : RelationalOperator  Operator===  OutDataTypeStr=boolean  RndMeth=Simplest
  Sum : Sum  Inputs=|+++
  Switch : Switch  Criteria=u2 > Threshold
  Switch1 : Switch  Criteria=u2 > Threshold
  Switch2 : Switch  Criteria=u2 > Threshold
  fall_set : Outport
  wires:
  Relational Operator/1 -> Switch/2
  Memory6/1 -> Relational Operator/2, Relational Operator2/2, Relational Operator1/2
  fall_signal/1 -> Relational Operator2/1, Relational Operator1/1, Relational Operator/1, Memory6/1
  Constant/1 -> Switch/1
  Constant1/1 -> Switch1/3, Switch/3
  Relational Operator1/1 -> Switch1/2
  Constant2/1 -> Switch1/1
  Constant3/1 -> Switch2/1
  Relational Operator2/1 -> Switch2/2
  Switch/1 -> Sum/1
  Switch1/1 -> Sum/2
  Switch2/1 -> Sum/3
  Sum/1 -> Multiport Switch/1
  Constant4/1 -> Multiport Switch/2
  Constant5/1 -> Multiport Switch/3
  Multiport Switch/1 -> fall_set/1, Memory/1
  Memory/1 -> Multiport Switch/4

== system teach_from_joints/traj_planing/joint_traj/joint_traj_sub/update_clock/Triggered Subsystem ==
  In1 : Inport
  Trigger : TriggerPort  VariantControl=Variant
  Out1 : Outport
  wires:
  In1/1 -> Out1/1

== system teach_from_joints/traj_planing/joint_traj/joint_traj_sub/update_clock/Triggered Subsystem1 ==
  In1 : Inport
  Trigger : TriggerPort  VariantControl=Variant
  Out1 : Outport
  wires:
  In1/1 -> Out1/1

== matlab function teach_from_joints/traj_function ==
  data: xyz output; rpy output; reach_count input; Px input; Py input; Pz input
function [xyz, rpy] = traj_function(reach_count,Px,Py,Pz)
    %base_xyz = [297.7,0,385.1];
    base_xyz = [274.5,0,405.1+0.4];%0.4：第一个SAMPLE_TIME后target需要有点改变
    base_rpy = [180,0,0];
    delta_xyz = [0,0,0];
    delta_rpy = [0,0,0];
    
%     delta_xyz(1) = Px(reach_count+1);
%     delta_xyz(2) = Py(reach_count+1);
%     delta_xyz(3) = Pz(reach_count+1);
    
    if reach_count == 1
        delta_xyz = [100,100,0];
        delta_rpy = [0,0,0];
    elseif reach_count == 2 || reach_count == 3
        delta_xyz = [-100,-100,0];
        delta_rpy = [0,0,0];
    end

    xyz = base_xyz + delta_xyz;
    rpy = base_rpy + delta_rpy;
end

== matlab function teach_from_joints/traj_planing/joint_traj/forward_kinematic/MATLAB Function ==
  data: theta input; T output; theta_offset input; d input; a input; alpha input
function T     = forward_kinematic_pack_modify( theta,theta_offset, d, a, alpha )
%DH_KINEMATIC input standard D_H parameter, output homogeneous matrix
%   
len = 6;
T_0_n = diag([1 1 1 1]);

for i = 1:len
    c_t = cos(theta(i) + theta_offset(i)); s_t = sin(theta(i) + theta_offset(i));
    c_a = cos(alpha(i)); s_a = sin(alpha(i));
    aa = a(i); dd =d(i);
    %homogeneous matrix between two link rods
    temp_T = [c_t       -s_t        0       aa
              s_t*c_a   c_t*c_a     -s_a    -dd*s_a
              s_t*s_a   c_t*s_a     c_a     dd*c_a
              0         0           0       1];
    %       
    T_0_n = T_0_n * temp_T;
end
   T = [1,0,0,0;0,1,0,0;0,0,1,0.3855+0.02;0,0,0,1]*T_0_n;
end

== matlab function teach_from_joints/traj_planing/joint_traj/forward_kinematic/MATLAB Function1 ==
  data: T input; xyzrpy output; last_rpy input
function xyzrpy    = matr2xyzrpy( T, last_rpy )
%通过齐次矩阵计算对应的位姿
%-pi/2 <= P <= pi; -pi/2 <= R <= pi; -pi <= P <= pi
%首先判断俯仰角P
xyzrpy = zeros(1, 6);% 用于存储x y z r(roll 翻滚角) p(pitch 俯仰角) y(yaw偏航角)
xyzrpy(1,1) = T(1, 4);% 获取x轴坐标
xyzrpy(1,2) = T(2, 4);% 获取y轴坐标
xyzrpy(1,3) = T(3, 4);% 获取z轴坐标
rpy = zeros(1, 3);
m = T(1:3, 1:3);
threshold = 1e-5;% 判断是否为0的阈值
max_change = 0.5;
for i = 1:3
    for j = 1:3
        if abs(m(i, j)) < threshold % 小于改阈值则为0
            m(i, j) = 0;
        end
    end
end
	% T = [ R，p；0，1 ]
	% 首先欧拉角定义（XYZ顺序）
	% 旋转顺序：先绕X轴转roll（φ），再绕Y轴转pitch（θ），最后绕Z轴转yaw（ψ）
	% 对应的旋转矩阵：R = Rx(φ) * Ry(θ) * Rz(ψ)
	% 展开：T =
	% [                               cos(pitch)*cos(yaw),                               -cos(pitch)*sin(yaw),            sin(pitch)]
	% [cos(roll)*sin(yaw) + cos(yaw)*sin(pitch)*sin(roll), cos(roll)*cos(yaw) - sin(pitch)*sin(roll)*sin(yaw), -	cos(pitch)*sin(roll)]
	% [sin(roll)*sin(yaw) - cos(roll)*cos(yaw)*sin(pitch), cos(yaw)*sin(roll) + cos(roll)*sin(pitch)*sin(yaw),  	cos(pitch)*cos(roll)]
	% 此处m = T
        if abs(m(3,3)) < threshold && abs(m(2,3)) < threshold	% 奇异情况-	cos(pitch)*sin(roll)和cos(pitch)*cos(roll)等于0,sin(pitch)>0,则pitch=pi/2
            % singularity
%             rpy(1) = 0;  % roll is zero
%             rpy(2) = atan2(m(1,3), m(3,3));  % pitch
%             rpy(3) = atan2(m(2,1), m(2,2));  % yaw is sum of roll+yaw
            if m(1, 3) > 0
                rpy(2) = pi/2;
		% R =[0,0,1;sin(roll+yaw),cos(roll+yaw),0;-cos(roll+yaw),sin(roll+yaw),0];
                temp_YandR = atan2(m(2,1), m(2,2));
                temp_last_YandR = last_rpy(3) + last_rpy(1);
                %%修正两个和的值，相差2*pi
                if temp_YandR > (temp_last_YandR + 2*max_change)
                    temp_YandR = temp_YandR - 2*pi;
                elseif temp_YandR < (temp_last_YandR - 2*max_change)
                    temp_YandR = temp_YandR + 2*pi;
                else
                    %
                end
                rpy(1) = last_rpy(1); 
                rpy(3) = temp_YandR - rpy(1);
                
                if rpy(3)> pi
                    rpy(3) = pi;
                elseif rpy(3)< -pi
                    rpy(3) = -pi;
                end
                    rpy(1) = temp_YandR - rpy(3);
            else
                rpy(2) = -pi/2;
		% R = [0,0,-1;sin(roll-yaw),cos(roll-yaw),0;cos(roll-yaw),-sin(roll-yaw),0];
                temp_YsbuR = atan2(m(2,1), m(2,2));
                temp_last_YsbuR = last_rpy(3) - last_rpy(1);
                if temp_YsbuR > (temp_last_YsbuR + 2*max_change)
                    temp_YsbuR = temp_YsbuR - 2*pi;
                elseif temp_YsbuR < (temp_last_YsbuR - 2*max_change)
                    temp_YsbuR = temp_YsbuR + 2*pi;
                else
                    %
                end
                rpy(1) = last_rpy(1); 
                rpy(3) = temp_YsbuR + rpy(1);
                
                %再修正一下Y值，防止它超出（-pi, pi),
                %这里实际上还是不能保证R和Y值是确定的，只是保证他们是连续的，而且再就是不要超出正常范围。
                if rpy(3)> pi
                    rpy(3) = pi;
                elseif rpy(3)< -pi
                    rpy(3) = -pi;
                end
                    rpy(1) = temp_YsbuR - rpy(3);
            end
            test = 1;    
        else
            %当P不等于正负pi/2时，非奇异情况
%             test = m(3,3)

            rpy(1) = atan2(-m(2,3), m(3,3));        % roll
            %rpy(1)等于正负pi时效果是一样的，取+pi更好，特别是相对初始零位关节5转动90度。
            if abs(rpy(1) - (-pi)) <= threshold
                rpy(1) = pi;
            end
            % compute sin/cos of roll angle
            sr = sin(rpy(1));
            cr = cos(rpy(1));
            rpy(2) = atan2(m(1,3), cr * m(3,3) - sr * m(2,3));  % pitch
            if abs(rpy(2)) < threshold	%（pitch在±90°附近）
                rpy(2) = last_rpy(2);
            end
            if cos(rpy(2)) > 0	%（pitch不在±90°附近）
                rpy(3) = atan2(-m(1,2), m(1,1));
            else
                rpy(3) = atan2(m(1,2), -m(1,1));
            end
            test = 2;  
        end

 xyzrpy(4:6) = rpy(1:3);
end

% function new_rpy1 = correct_ryy1(ryp1)
%     if ryp1 > pi
%         new_rpy1 = ryp1 - pi
% 
% end




%%
% test
% syms C_R S_R C_P S_P C_Y S_Y
%  rotate_x = [1       0       0
%                 0       C_R     -S_R
%                 0       S_R     C_R];  
% 
%     rotate_y = [C_P     0       S_P
%                 0       1       0
%                 -S_P    0       C_P];  
%             
%     rotate_z = [C_Y     -S_Y	0
%                 S_Y     C_Y     0
%                 0       0       1];  
% M = rotate_x * rotate_y * rotate_z
%  
% M =+
% [               C_P*C_Y,              -C_P*S_Y,      S_P]
% [ C_R*S_Y + C_Y*S_P*S_R, C_R*C_Y - S_P*S_R*S_Y, -C_P*S_R]
% [ S_R*S_Y - C_R*C_Y*S_P, C_Y*S_R + C_R*S_P*S_Y,  C_P*C_R]
